simulink model "P1_Part2_Option1 (2)"  (R2023b)
settings: Solver=VariableStepAuto  StartTime=0.0  StopTime=25  RelTol=1e-3
values from neighbouring files (symbols this model uses):
  b1 = 1    [Project1_Part2.m]
  b2 = 1    [Project1_Part2.m]
  J1 = 100    [Project1_Part2.m]
  J2 = 1    [Project1_Part2.m]
  k = index5    [Project1_Part2.m]
  T_app = index1    [Project1_Part2.m]
settings Model: Creator=luker  LastModifiedBy=luker

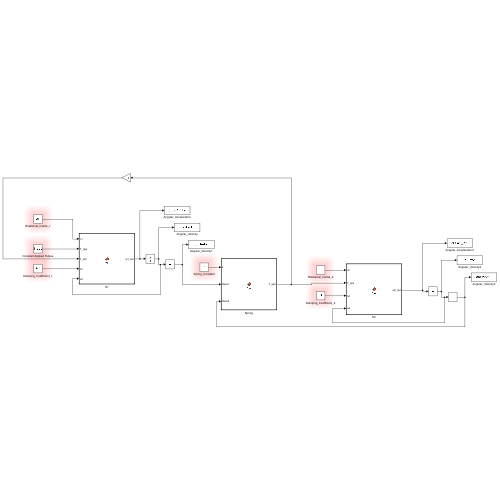
[thumbnail: Simulink's stored preview of the top-level diagram]
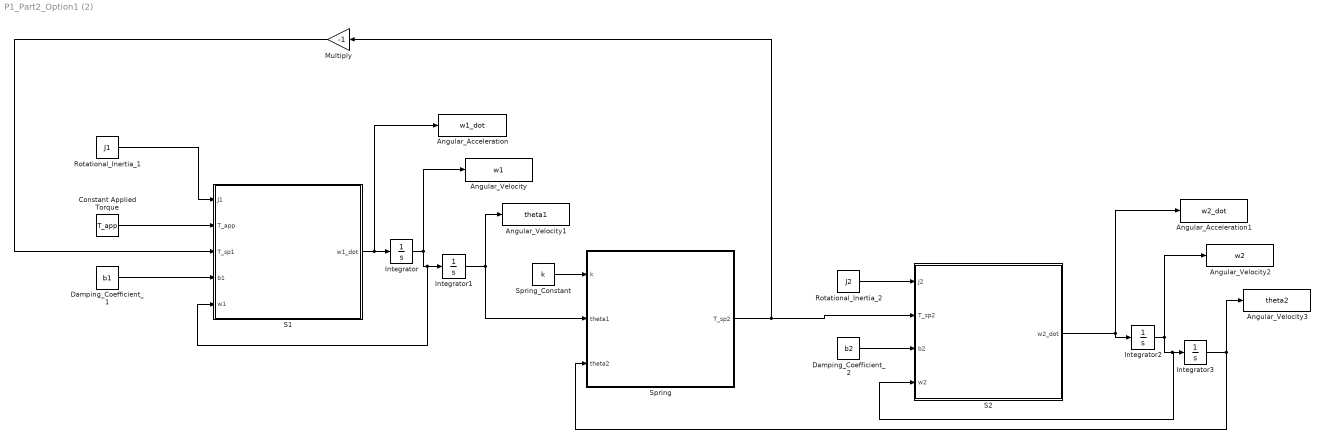
== system P1_Part2_Option1 (2) ==
  Angular_Acceleration : ToWorkspace  VariableName=w1_dot  SaveFormat=Timeseries  SampleTime=-1
  Angular_Acceleration1 : ToWorkspace  VariableName=w2_dot  SaveFormat=Timeseries  SampleTime=-1
  Angular_Velocity : ToWorkspace  VariableName=w1  SaveFormat=Timeseries  SampleTime=-1
  Angular_Velocity1 : ToWorkspace  VariableName=theta1  SaveFormat=Timeseries  SampleTime=-1
  Angular_Velocity2 : ToWorkspace  VariableName=w2  SaveFormat=Timeseries  SampleTime=-1
  Angular_Velocity3 : ToWorkspace  VariableName=theta2  SaveFormat=Timeseries  SampleTime=-1
  Constant Applied Torque : Constant  Value=T_app
  Damping_Coefficient_1 : Constant  Value=b1
  Damping_Coefficient_2 : Constant  Value=b2
  Integrator{,1..3} (4 alike) : Integrator  UpperSaturationLimit=<binary blob, 304 chars, not shown>  LowerSaturationLimit=<binary blob, 305 chars, not shown>
  Multiply : Gain  Gain=-1
  Rotational_Inertia_1 : Constant  Value=J1
  Rotational_Inertia_2 : Constant  Value=J2
  S1 : MATLAB Function  TreatAsAtomicUnit=on
  S2 : MATLAB Function  TreatAsAtomicUnit=on
  Spring : MATLAB Function  TreatAsAtomicUnit=on
  Spring_Constant : Constant  Value=k
  wires:
  Rotational_Inertia_1/1 -> S1/1(J1)
  Integrator/1 -> S1/5(w1), Integrator1/1, Angular_Velocity/1
  S1/1(w1_dot) -> Angular_Acceleration/1, Integrator/1
  Integrator1/1 -> Angular_Velocity1/1, Spring/2(theta1)
  Spring/1(T_sp2) -> Multiply/1, S2/2(T_sp2)
  Integrator2/1 -> S2/4(w2), Integrator3/1, Angular_Velocity2/1
  S2/1(w2_dot) -> Integrator2/1, Angular_Acceleration1/1
  Integrator3/1 -> Spring/3(theta2), Angular_Velocity3/1
  Multiply/1 -> S1/3(T_sp1)
  Damping_Coefficient_1/1 -> S1/4(b1)
  Constant Applied Torque/1 -> S1/2(T_app)
  Spring_Constant/1 -> Spring/1(k)
  Rotational_Inertia_2/1 -> S2/1(J2)
  Damping_Coefficient_2/1 -> S2/3(b2)

== matlab function P1_Part2_Option1 (2)/S2 ==
  data: J2 input; w2_dot output; T_sp2 input; b2 input; w2 input
function w2_dot = fcn(J2, T_sp2, b2, w2)
% GIVENS:
% J1
% B1
% J2
% B2
% T_app - Constant Applied Torque
% FOR OPTION 1:
% k

w2_dot = (1/J2)*(T_sp2-b2*w2);
end

== matlab function P1_Part2_Option1 (2)/S1 ==
  data: J1 input; w1_dot output; T_app input; T_sp1 input; b1 input; w1 input
function w1_dot = fcn(J1, T_app, T_sp1, b1, w1)
% GIVENS:
% J1
% B1
% J2
% B2
% T_app - Constant Applied Torque
% FOR OPTION 1:
% k

w1_dot = (1/J1)*(T_app-T_sp1-b1*w1);
end

== matlab function P1_Part2_Option1 (2)/Spring ==
  data: k input; T_sp2 output; theta1 input; theta2 input
function T_sp2 = fcn(k, theta1, theta2)
% GIVENS:
% J1
% B1
% J2
% B2
% T_app - Constant Applied Torque
% FOR OPTION 1:
% k

T_sp2 = (k)*(theta1-theta2);
end
